simulink model "sampleModel7293_pp_1_1"  (R2018a)
settings: Solver=VariableStepAuto  StartTime=0.0  StopTime=10.0  RelTol=1e-3
undefined symbols (not defined in the file): DiscIntNeverNeededParam
libraries: simulink x367
(part 11 of 12)

== system sampleModel7293_pp_1_1/cfblk210/cfblk18 ==
  cfblk1 : Inport
  cfblk12 : Inport  Port=2
  cfblk13 : Inport  Port=3
  Action Port : ActionPort  ActionType=else
  cfblk10 : simulink/Discrete/Transfer Fcn First Order  PoleZ=0.95  ICPrevOutput=0.0  DoSatur=off
      settings: SourceProductName=Simulink
  cfblk11 : UnitDelay  SampleTime=-1
  cfblk3 : simulink/Discrete/Transfer Fcn Real Zero  ZeroZ=0.75  ICPrevInput=0.0  DoSatur=off
      settings: SourceProductName=Simulink  SourceProductBaseCode=SL
  cfblk4 : Subsystem  TreatAsAtomicUnit=on
  cfblk5 : DiscreteIntegrator  SampleTime=-1  OutDataTypeStr=double  ICPrevOutput=DiscIntNeverNeededParam  ICPrevScaledInput=DiscIntNeverNeededParam
  cfblk6 : DiscreteZeroPole  Poles=[0 0.5]  Gain=1  SampleTime=-1
  cfblk7 : DiscreteFir
  cfblk8 : UnitDelay  SampleTime=-1
  cfblk9 : Subsystem  TreatAsAtomicUnit=on
  cyemi_{1386..1394} (9 alike) : DataTypeConversion  OutDataTypeStr=double
  emi_1581 : Subsystem  TreatAsAtomicUnit=on
  emi_1583 : If  IfExpression=0 <= u1
  emi_1584 : DataTypeConversion  OutDataTypeStr=double
  emi_1688 : Subsystem  TreatAsAtomicUnit=on
  emi_1690 : If  IfExpression=0 <= u1
  emi_1691 : DataTypeConversion  OutDataTypeStr=double
  cfblk2 : Outport
  wires:
  cfblk3/1 -> cfblk2/1
  cyemi_1386/1 -> cfblk10/1
  cfblk5/1 -> cyemi_1386/1, emi_1584/1
  cyemi_1387/1 -> cfblk11/1
  cfblk8/1 -> cyemi_1387/1, emi_1691/1
  cyemi_1388/1 -> cfblk3/1
  cfblk13/1 -> cyemi_1388/1
  cyemi_1390/1 -> cfblk5/1
  cfblk11/1 -> cyemi_1390/1
  cyemi_1391/1 -> cfblk6/1
  cfblk12/1 -> cyemi_1391/1
  cyemi_1392/1 -> cfblk7/1
  cfblk1/1 -> cyemi_1392/1
  cyemi_1393/1 -> cfblk8/1
  cfblk6/1 -> cyemi_1394/1
  cyemi_1389/1 -> cfblk4/1(emi_1579)
  cfblk4/1(emi_1580) -> cyemi_1393/1
  emi_1583/1 -> cfblk4/Action
  emi_1583/2 -> emi_1581/Action
  emi_1584/1 -> emi_1583/1
  cyemi_1394/1 -> cfblk9/1(emi_1686)
  cfblk9/1(emi_1687) -> cyemi_1389/1
  emi_1690/1 -> cfblk9/Action
  emi_1690/2 -> emi_1688/Action
  emi_1691/1 -> emi_1690/1

== system sampleModel7293_pp_1_1/cfblk211/cfblk5 ==
  emi_1857 : Inport
  Action Port : ActionPort  ActionType=then
  cfblk5 : simulink/Discrete/Transfer Fcn First Order  PoleZ=0.95  ICPrevOutput=0.0  DoSatur=off
      settings: SourceProductName=Simulink
  emi_1858 : Outport
  wires:
  emi_1857/1 -> cfblk5/1
  cfblk5/1 -> emi_1858/1

== system sampleModel7293_pp_1_1/cfblk211/emi_1859 ==
  Action Port : ActionPort  ActionType=else
  emi_1860 : Assertion

== system sampleModel7293_pp_1_1/cfblk213/cfblk10 ==
  emi_1330 : Inport
  Action Port : ActionPort  ActionType=then
  cfblk10 : DiscreteFir
  emi_1331 : Outport
  wires:
  emi_1330/1 -> cfblk10/1
  cfblk10/1 -> emi_1331/1

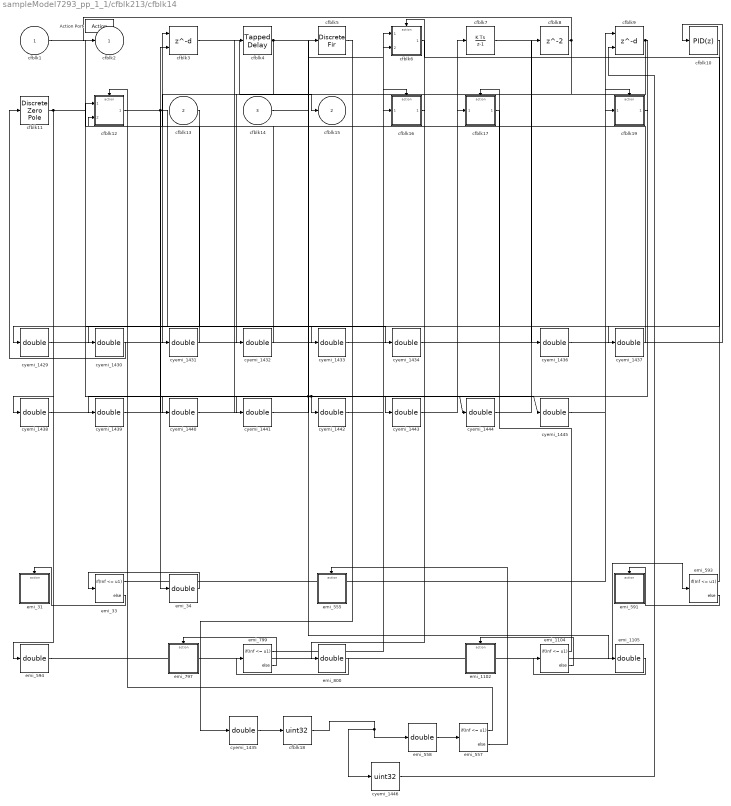
== system sampleModel7293_pp_1_1/cfblk213/cfblk14 ==
  cfblk1 : Inport
  cfblk13 : Inport  Port=2
  cfblk14 : Inport  Port=3
  Action Port : ActionPort  ActionType=then
  cfblk10 : simulink/Continuous/PID Controller  Controller=PID  TimeDomain=Discrete-time  SampleTime=-1  IntegratorMethod=Forward Euler  FilterMethod=Forward Euler  Form=Parallel  UseFilter=on  ControllerParametersSource=internal  P=1  I=1  D=0  N=100  InitialConditionSource=internal  InitialConditionForIntegrator=0  InitialConditionForFilter=0  ExternalReset=none  LimitOutput=off  UpperSaturationLimit=inf  LowerSaturationLimit=-inf  LinearizeAsGain=off  AntiWindupMode=none  Kb=1  TrackingMode=off  Kt=1  PParamMin=[]  PParamMax=[]  IParamMin=[]  IParamMax=[]  DParamMin=[]  DParamMax=[]  NParamMin=[]  NParamMax=[]  KbParamMin=[]  KbParamMax=[]  KtParamMin=[]  KtParamMax=[]  POutMin=[]  POutMax=[]  IOutMin=[]  IOutMax=[]  DOutMin=[]  DOutMax=[]  NOutMin=[]  NOutMax=[]  KbOutMin=[]  KbOutMax=[]  KtOutMin=[]  KtOutMax=[]  IntegratorOutMin=[]  IntegratorOutMax=[]  FilterOutMin=[]  FilterOutMax=[]  SumOutMin=[]  SumOutMax=[]  SumI1OutMin=[]  SumI1OutMax=[]  SumI2OutMin=[]  SumI2OutMax=[]  SumI3OutMin=[]  SumI3OutMax=[]  SumDOutMin=[]  SumDOutMax=[]  SaturationOutMin=[]  SaturationOutMax=[]  IntegratorContinuousStateAttributes=''  IntegratorStateMustResolveToSignalObject=off  IntegratorRTWStateStorageClass=Auto  FilterContinuousStateAttributes=''  FilterStateMustResolveToSignalObject=off  FilterRTWStateStorageClass=Auto  DifferentiatorICPrevScaledInput=0  DifferentiatorOutMin=[]  DifferentiatorOutMax=[]  FilterDiffOutCoefMin=[]  FilterDiffOutCoefMax=[]  SumDenOutMin=[]  SumDenOutMax=[]  SumNumOutMin=[]  SumNumOutMax=[]  ReciprocalOutMin=[]  ReciprocalOutMax=[]  DivideOutMin=[]  DivideOutMax=[]  TunerSelectOption=Transfer Function Based (PID Tuner App)
  cfblk11 : DiscreteZeroPole  Poles=[0 0.5]  Gain=1  SampleTime=-1
  cfblk12 : Subsystem  TreatAsAtomicUnit=on
  cfblk16 : Subsystem  TreatAsAtomicUnit=on
  cfblk17 : Subsystem  TreatAsAtomicUnit=on
  cfblk18 : DataTypeConversion  OutDataTypeStr=uint32
  cfblk19 : Subsystem  TreatAsAtomicUnit=on
  cfblk3 : Delay  DelayLengthSource=Input port
      settings: InputPortMap=u0,p1
  cfblk4 : simulink/Discrete/Tapped Delay  vinit=0.0  samptime=-1  NumDelays=1  DelayOrder=Oldest  includeCurrent=off
  cfblk5 : DiscreteFir
  cfblk6 : Subsystem  TreatAsAtomicUnit=on
  cfblk7 : DiscreteIntegrator  SampleTime=-1  OutDataTypeStr=double  ICPrevOutput=DiscIntNeverNeededParam  ICPrevScaledInput=DiscIntNeverNeededParam
  cfblk8 : Delay
  cfblk9 : Delay  DelayLengthSource=Input port
      settings: InputPortMap=u0,p1
  cyemi_{1429..1445} (17 alike) : DataTypeConversion  OutDataTypeStr=double
  cyemi_1446 : DataTypeConversion  OutDataTypeStr=uint32
  emi_1102 : Subsystem  TreatAsAtomicUnit=on
  emi_{33,557,593,799,1104} (5 alike) : If  IfExpression=Inf <= u1
  emi_{34,558,594,800,1105} (5 alike) : DataTypeConversion  OutDataTypeStr=double
  emi_31 : Subsystem  TreatAsAtomicUnit=on
  emi_555 : Subsystem  TreatAsAtomicUnit=on
  emi_591 : Subsystem  TreatAsAtomicUnit=on
  emi_797 : Subsystem  TreatAsAtomicUnit=on
  cfblk2 : Outport
  cfblk15 : Outport  Port=2
  wires:
  cfblk3/1 -> cfblk15/1
  cfblk8/1 -> cfblk2/1, emi_800/1
  cfblk1/1 -> cyemi_1442/1, cyemi_1444/1
  cfblk4/1 -> cyemi_1445/1, emi_1105/1, cyemi_1431/1
  cfblk9/1 -> cyemi_1432/1, cyemi_1437/1
  cyemi_1429/1 -> cfblk10/1
  cyemi_1430/1 -> cfblk11/1
  cfblk10/1 -> cyemi_1430/1
  cfblk11/1 -> cyemi_1434/1, emi_594/1
  cyemi_1435/1 -> cfblk18/1
  cfblk5/1 -> cyemi_1435/1
  cfblk7/1 -> cyemi_1436/1
  cyemi_1437/1 -> cfblk3/1
  cyemi_1438/1 -> cfblk3/2
  cfblk13/1 -> cyemi_1438/1
  cyemi_1439/1 -> cfblk4/1
  cyemi_1440/1 -> cfblk5/1
  cyemi_1443/1 -> cfblk7/1
  cfblk14/1 -> cyemi_1443/1
  cyemi_1444/1 -> cfblk8/1
  cyemi_1445/1 -> cfblk9/1
  cyemi_1446/1 -> cfblk9/2
  cfblk18/1 -> emi_558/1, cyemi_1446/1
  cyemi_1436/1 -> cfblk19/1(emi_29)
  cfblk19/1(emi_30) -> cyemi_1440/1
  emi_33/1 -> cfblk19/Action
  emi_33/2 -> emi_31/Action
  emi_34/1 -> emi_33/1
  cyemi_1431/1 -> cfblk12/1(emi_552)
  cyemi_1432/1 -> cfblk12/2(emi_553)
  cfblk12/1(emi_554) -> emi_34/1, cyemi_1433/1
  emi_557/1 -> cfblk12/Action
  emi_557/2 -> emi_555/Action
  emi_558/1 -> emi_557/1
  cyemi_1441/1 -> cfblk6/1(emi_588)
  cyemi_1442/1 -> cfblk6/2(emi_589)
  cfblk6/1(emi_590) -> cyemi_1439/1
  emi_593/1 -> cfblk6/Action
  emi_593/2 -> emi_591/Action
  emi_594/1 -> emi_593/1
  cyemi_1433/1 -> cfblk16/1(emi_795)
  cfblk16/1(emi_796) -> cyemi_1441/1
  emi_799/1 -> cfblk16/Action
  emi_799/2 -> emi_797/Action
  emi_800/1 -> emi_799/1
  cyemi_1434/1 -> cfblk17/1(emi_1100)
  cfblk17/1(emi_1101) -> cyemi_1429/1
  emi_1104/1 -> cfblk17/Action
  emi_1104/2 -> emi_1102/Action
  emi_1105/1 -> emi_1104/1

== system sampleModel7293_pp_1_1/cfblk213/cfblk15 ==
  cfblk1 : Inport
  cfblk9 : Inport  Port=2
  Action Port : ActionPort  ActionType=else
  cfblk11 : Delay
  cfblk12 : Delay
  cfblk3 : DiscreteIntegrator  SampleTime=-1  OutDataTypeStr=double  ICPrevOutput=DiscIntNeverNeededParam  ICPrevScaledInput=DiscIntNeverNeededParam
  cfblk4 : UnitDelay  SampleTime=-1
  cfblk5 : Delay
  cfblk6 : UnitDelay  SampleTime=-1
  cfblk7 : simulink/Discrete/Tapped Delay  vinit=0.0  samptime=-1  NumDelays=1  DelayOrder=Oldest  includeCurrent=off
  cfblk8 : DiscreteZeroPole  Poles=[0 0.5]  Gain=1  SampleTime=-1
  cyemi_{1449..1456} (8 alike) : DataTypeConversion  OutDataTypeStr=double
  cfblk2 : Outport
  cfblk10 : Outport  Port=2
  wires:
  cfblk1/1 -> cfblk10/1
  cfblk8/1 -> cfblk2/1
  cyemi_1449/1 -> cfblk11/1
  cfblk6/1 -> cyemi_1449/1
  cyemi_1450/1 -> cfblk12/1
  cfblk5/1 -> cyemi_1450/1
  cyemi_1451/1 -> cfblk3/1
  cfblk11/1 -> cyemi_1451/1
  cyemi_1452/1 -> cfblk4/1
  cfblk12/1 -> cyemi_1452/1
  cyemi_1453/1 -> cfblk5/1
  cfblk4/1 -> cyemi_1453/1
  cyemi_1454/1 -> cfblk6/1
  cfblk3/1 -> cyemi_1454/1
  cyemi_1455/1 -> cfblk7/1
  cfblk9/1 -> cyemi_1455/1
  cyemi_1456/1 -> cfblk8/1
  cfblk7/1 -> cyemi_1456/1

== system sampleModel7293_pp_1_1/cfblk213/cfblk16 ==
  emi_1358 : Inport
  Action Port : ActionPort  ActionType=then
  cfblk16 : Delay
  emi_1359 : Outport
  wires:
  emi_1358/1 -> cfblk16/1
  cfblk16/1 -> emi_1359/1

== system sampleModel7293_pp_1_1/cfblk213/emi_1332 ==
  Action Port : ActionPort  ActionType=else
  emi_1333 : Assertion

== system sampleModel7293_pp_1_1/cfblk213/emi_1360 ==
  Action Port : ActionPort  ActionType=else
  emi_1361 : Assertion

== system sampleModel7293_pp_1_1/cfblk165/cfblk15/cfblk11 ==
  emi_1022 : Inport
  Action Port : ActionPort  ActionType=then
  cfblk11 : DiscreteFir
  emi_1023 : Outport
  wires:
  emi_1022/1 -> cfblk11/1
  cfblk11/1 -> emi_1023/1

== system sampleModel7293_pp_1_1/cfblk165/cfblk15/cfblk12 ==
  emi_1408 : Inport
  Action Port : ActionPort  ActionType=then
  cfblk12 : Delay
  emi_1409 : Outport
  wires:
  emi_1408/1 -> cfblk12/1
  cfblk12/1 -> emi_1409/1

== system sampleModel7293_pp_1_1/cfblk165/cfblk15/cfblk13 ==
  emi_1764 : Inport
  Action Port : ActionPort  ActionType=then
  cfblk13 : DiscreteStateSpace  SampleTime=-1
  emi_1765 : Outport
  wires:
  emi_1764/1 -> cfblk13/1
  cfblk13/1 -> emi_1765/1

== system sampleModel7293_pp_1_1/cfblk165/cfblk15/emi_1024 ==
  Action Port : ActionPort  ActionType=else
  emi_1025 : Assertion

== system sampleModel7293_pp_1_1/cfblk165/cfblk15/emi_1410 ==
  Action Port : ActionPort  ActionType=else
  emi_1411 : Assertion

== system sampleModel7293_pp_1_1/cfblk165/cfblk15/emi_1766 ==
  Action Port : ActionPort  ActionType=else
  emi_1767 : Assertion

== system sampleModel7293_pp_1_1/cfblk165/cfblk16/cfblk11 ==
  emi_150 : Inport
  Action Port : ActionPort  ActionType=then
  cfblk11 : simulink/Discrete/Transfer Fcn Real Zero  ZeroZ=0.75  ICPrevInput=0.0  DoSatur=off
      settings: SourceProductName=Simulink  SourceProductBaseCode=SL
  emi_151 : Outport
  wires:
  emi_150/1 -> cfblk11/1
  cfblk11/1 -> emi_151/1

== system sampleModel7293_pp_1_1/cfblk165/cfblk16/cfblk12 ==
  emi_1157 : Inport
  emi_1158 : Inport  Port=2
  Action Port : ActionPort  ActionType=then
  cfblk12 : Delay  ShowEnablePort=on
      settings: InputPortMap=u0,e6
  emi_1159 : Outport
  wires:
  emi_1157/1 -> cfblk12/1
  emi_1158/1 -> cfblk12/2
  cfblk12/1 -> emi_1159/1

== system sampleModel7293_pp_1_1/cfblk165/cfblk16/cfblk8 ==
  emi_2075 : Inport
  Action Port : ActionPort  ActionType=then
  cfblk8 : UnitDelay  SampleTime=-1
  emi_2076 : Outport
  wires:
  emi_2075/1 -> cfblk8/1
  cfblk8/1 -> emi_2076/1

== system sampleModel7293_pp_1_1/cfblk165/cfblk16/emi_1160 ==
  Action Port : ActionPort  ActionType=else
  emi_1161 : Assertion

== system sampleModel7293_pp_1_1/cfblk165/cfblk16/emi_152 ==
  Action Port : ActionPort  ActionType=else
  emi_153 : Assertion

== system sampleModel7293_pp_1_1/cfblk165/cfblk16/emi_2077 ==
  Action Port : ActionPort  ActionType=else
  emi_2078 : Assertion

== system sampleModel7293_pp_1_1/cfblk167/cfblk17/cfblk5 ==
  emi_415 : Inport
  Action Port : ActionPort  ActionType=then
  cfblk5 : simulink/Discrete/Transfer Fcn Real Zero  ZeroZ=0.75  ICPrevInput=0.0  DoSatur=off
      settings: SourceProductName=Simulink  SourceProductBaseCode=SL
  emi_416 : Outport
  wires:
  emi_415/1 -> cfblk5/1
  cfblk5/1 -> emi_416/1

== system sampleModel7293_pp_1_1/cfblk167/cfblk17/cfblk7 ==
  emi_531 : Inport
  Action Port : ActionPort  ActionType=then
  cfblk7 : simulink/Continuous/PID Controller  Controller=PID  TimeDomain=Discrete-time  SampleTime=-1  IntegratorMethod=Forward Euler  FilterMethod=Forward Euler  Form=Parallel  UseFilter=on  ControllerParametersSource=internal  P=1  I=1  D=0  N=100  InitialConditionSource=internal  InitialConditionForIntegrator=0  InitialConditionForFilter=0  ExternalReset=none  LimitOutput=off  UpperSaturationLimit=inf  LowerSaturationLimit=-inf  LinearizeAsGain=off  AntiWindupMode=none  Kb=1  TrackingMode=off  Kt=1  PParamMin=[]  PParamMax=[]  IParamMin=[]  IParamMax=[]  DParamMin=[]  DParamMax=[]  NParamMin=[]  NParamMax=[]  KbParamMin=[]  KbParamMax=[]  KtParamMin=[]  KtParamMax=[]  POutMin=[]  POutMax=[]  IOutMin=[]  IOutMax=[]  DOutMin=[]  DOutMax=[]  NOutMin=[]  NOutMax=[]  KbOutMin=[]  KbOutMax=[]  KtOutMin=[]  KtOutMax=[]  IntegratorOutMin=[]  IntegratorOutMax=[]  FilterOutMin=[]  FilterOutMax=[]  SumOutMin=[]  SumOutMax=[]  SumI1OutMin=[]  SumI1OutMax=[]  SumI2OutMin=[]  SumI2OutMax=[]  SumI3OutMin=[]  SumI3OutMax=[]  SumDOutMin=[]  SumDOutMax=[]  SaturationOutMin=[]  SaturationOutMax=[]  IntegratorContinuousStateAttributes=''  IntegratorStateMustResolveToSignalObject=off  IntegratorRTWStateStorageClass=Auto  FilterContinuousStateAttributes=''  FilterStateMustResolveToSignalObject=off  FilterRTWStateStorageClass=Auto  DifferentiatorICPrevScaledInput=0  DifferentiatorOutMin=[]  DifferentiatorOutMax=[]  FilterDiffOutCoefMin=[]  FilterDiffOutCoefMax=[]  SumDenOutMin=[]  SumDenOutMax=[]  SumNumOutMin=[]  SumNumOutMax=[]  ReciprocalOutMin=[]  ReciprocalOutMax=[]  DivideOutMin=[]  DivideOutMax=[]  TunerSelectOption=Transfer Function Based (PID Tuner App)
  emi_532 : Outport
  wires:
  emi_531/1 -> cfblk7/1
  cfblk7/1 -> emi_532/1

== system sampleModel7293_pp_1_1/cfblk167/cfblk17/emi_417 ==
  Action Port : ActionPort  ActionType=else
  emi_418 : Assertion

== system sampleModel7293_pp_1_1/cfblk167/cfblk17/emi_533 ==
  Action Port : ActionPort  ActionType=else
  emi_534 : Assertion

== system sampleModel7293_pp_1_1/cfblk167/cfblk18/cfblk4 ==
  emi_1557 : Inport
  Action Port : ActionPort  ActionType=then
  cfblk4 : DiscreteZeroPole  Poles=[0 0.5]  Gain=1  SampleTime=-1
  emi_1558 : Outport
  wires:
  emi_1557/1 -> cfblk4/1
  cfblk4/1 -> emi_1558/1

== system sampleModel7293_pp_1_1/cfblk167/cfblk18/cfblk6 ==
  emi_2119 : Inport
  Action Port : ActionPort  ActionType=then
  cfblk6 : simulink/Discrete/Transfer Fcn Real Zero  ZeroZ=0.75  ICPrevInput=0.0  DoSatur=off
      settings: SourceProductName=Simulink  SourceProductBaseCode=SL
  emi_2120 : Outport
  wires:
  emi_2119/1 -> cfblk6/1
  cfblk6/1 -> emi_2120/1

== system sampleModel7293_pp_1_1/cfblk167/cfblk18/cfblk8 ==
  emi_36 : Inport
  Action Port : ActionPort  ActionType=then
  cfblk8 : DiscreteTransferFcn
  emi_37 : Outport
  wires:
  emi_36/1 -> cfblk8/1
  cfblk8/1 -> emi_37/1

== system sampleModel7293_pp_1_1/cfblk167/cfblk18/emi_1559 ==
  Action Port : ActionPort  ActionType=else
  emi_1560 : Assertion

== system sampleModel7293_pp_1_1/cfblk167/cfblk18/emi_2121 ==
  Action Port : ActionPort  ActionType=else
  emi_2122 : Assertion

== system sampleModel7293_pp_1_1/cfblk167/cfblk18/emi_38 ==
  Action Port : ActionPort  ActionType=else
  emi_39 : Assertion

== system sampleModel7293_pp_1_1/cfblk167/cfblk20/cfblk5 ==
  emi_72 : Inport
  Action Port : ActionPort  ActionType=then
  cfblk5 : simulink/Continuous/PID Controller  Controller=PID  TimeDomain=Discrete-time  SampleTime=-1  IntegratorMethod=Forward Euler  FilterMethod=Forward Euler  Form=Parallel  UseFilter=on  ControllerParametersSource=internal  P=1  I=1  D=0  N=100  InitialConditionSource=internal  InitialConditionForIntegrator=0  InitialConditionForFilter=0  ExternalReset=none  LimitOutput=off  UpperSaturationLimit=inf  LowerSaturationLimit=-inf  LinearizeAsGain=off  AntiWindupMode=none  Kb=1  TrackingMode=off  Kt=1  PParamMin=[]  PParamMax=[]  IParamMin=[]  IParamMax=[]  DParamMin=[]  DParamMax=[]  NParamMin=[]  NParamMax=[]  KbParamMin=[]  KbParamMax=[]  KtParamMin=[]  KtParamMax=[]  POutMin=[]  POutMax=[]  IOutMin=[]  IOutMax=[]  DOutMin=[]  DOutMax=[]  NOutMin=[]  NOutMax=[]  KbOutMin=[]  KbOutMax=[]  KtOutMin=[]  KtOutMax=[]  IntegratorOutMin=[]  IntegratorOutMax=[]  FilterOutMin=[]  FilterOutMax=[]  SumOutMin=[]  SumOutMax=[]  SumI1OutMin=[]  SumI1OutMax=[]  SumI2OutMin=[]  SumI2OutMax=[]  SumI3OutMin=[]  SumI3OutMax=[]  SumDOutMin=[]  SumDOutMax=[]  SaturationOutMin=[]  SaturationOutMax=[]  IntegratorContinuousStateAttributes=''  IntegratorStateMustResolveToSignalObject=off  IntegratorRTWStateStorageClass=Auto  FilterContinuousStateAttributes=''  FilterStateMustResolveToSignalObject=off  FilterRTWStateStorageClass=Auto  DifferentiatorICPrevScaledInput=0  DifferentiatorOutMin=[]  DifferentiatorOutMax=[]  FilterDiffOutCoefMin=[]  FilterDiffOutCoefMax=[]  SumDenOutMin=[]  SumDenOutMax=[]  SumNumOutMin=[]  SumNumOutMax=[]  ReciprocalOutMin=[]  ReciprocalOutMax=[]  DivideOutMin=[]  DivideOutMax=[]  TunerSelectOption=Transfer Function Based (PID Tuner App)
  emi_73 : Outport
  wires:
  emi_72/1 -> cfblk5/1
  cfblk5/1 -> emi_73/1

== system sampleModel7293_pp_1_1/cfblk167/cfblk20/cfblk8 ==
  emi_250 : Inport
  Action Port : ActionPort  ActionType=then
  cfblk8 : Delay
  emi_251 : Outport
  wires:
  emi_250/1 -> cfblk8/1
  cfblk8/1 -> emi_251/1

== system sampleModel7293_pp_1_1/cfblk167/cfblk20/emi_252 ==
  Action Port : ActionPort  ActionType=else
  emi_253 : Assertion

== system sampleModel7293_pp_1_1/cfblk167/cfblk20/emi_74 ==
  Action Port : ActionPort  ActionType=else
  emi_75 : Assertion

== system sampleModel7293_pp_1_1/cfblk170/cfblk14/cfblk5 ==
  emi_1664 : Inport
  emi_1665 : Inport  Port=2
  Action Port : ActionPort  ActionType=then
  cfblk5 : Delay  ShowEnablePort=on
      settings: InputPortMap=u0,e6
  emi_1666 : Outport
  wires:
  emi_1664/1 -> cfblk5/1
  emi_1665/1 -> cfblk5/2
  cfblk5/1 -> emi_1666/1

== system sampleModel7293_pp_1_1/cfblk170/cfblk14/cfblk8 ==
  emi_667 : Inport
  Action Port : ActionPort  ActionType=then
  cfblk8 : Delay
  emi_668 : Outport
  wires:
  emi_667/1 -> cfblk8/1
  cfblk8/1 -> emi_668/1

== system sampleModel7293_pp_1_1/cfblk170/cfblk14/emi_1667 ==
  Action Port : ActionPort  ActionType=else
  emi_1668 : Assertion

== system sampleModel7293_pp_1_1/cfblk170/cfblk14/emi_669 ==
  Action Port : ActionPort  ActionType=else
  emi_670 : Assertion

== system sampleModel7293_pp_1_1/cfblk170/cfblk15/cfblk4 ==
  emi_1864 : Inport
  Action Port : ActionPort  ActionType=then
  cfblk4 : DiscreteFir
  emi_1865 : Outport
  wires:
  emi_1864/1 -> cfblk4/1
  cfblk4/1 -> emi_1865/1

== system sampleModel7293_pp_1_1/cfblk170/cfblk15/cfblk5 ==
  emi_1843 : Inport
  Action Port : ActionPort  ActionType=then
  cfblk5 : Delay
  emi_1844 : Outport
  wires:
  emi_1843/1 -> cfblk5/1
  cfblk5/1 -> emi_1844/1

== system sampleModel7293_pp_1_1/cfblk170/cfblk15/cfblk7 ==
  emi_185 : Inport
  emi_186 : Inport  Port=2
  Action Port : ActionPort  ActionType=then
  cfblk7 : simulink/Continuous/PID Controller (2DOF)  Controller=PID  TimeDomain=Discrete-time  SampleTime=-1  IntegratorMethod=Forward Euler  FilterMethod=Forward Euler  Form=Parallel  UseFilter=on  ControllerParametersSource=internal  P=1  I=1  D=0  N=100  b=1  c=1  InitialConditionSource=internal  InitialConditionForIntegrator=0  InitialConditionForFilter=0  ExternalReset=none  LimitOutput=off  UpperSaturationLimit=inf  LowerSaturationLimit=-inf  LinearizeAsGain=off  AntiWindupMode=none  Kb=1  TrackingMode=off  Kt=1  PParamMin=[]  PParamMax=[]  IParamMin=[]  IParamMax=[]  DParamMin=[]  DParamMax=[]  NParamMin=[]  NParamMax=[]  bParamMin=[]  bParamMax=[]  cParamMin=[]  cParamMax=[]  KbParamMin=[]  KbParamMax=[]  KtParamMin=[]  KtParamMax=[]  POutMin=[]  POutMax=[]  IOutMin=[]  IOutMax=[]  DOutMin=[]  DOutMax=[]  NOutMin=[]  NOutMax=[]  bOutMin=[]  bOutMax=[]  cOutMin=[]  cOutMax=[]  KbOutMin=[]  KbOutMax=[]  KtOutMin=[]  KtOutMax=[]  IntegratorOutMin=[]  IntegratorOutMax=[]  FilterOutMin=[]  FilterOutMax=[]  SumOutMin=[]  SumOutMax=[]  Sum1OutMin=[]  Sum1OutMax=[]  Sum2OutMin=[]  Sum2OutMax=[]  Sum3OutMin=[]  Sum3OutMax=[]  SumI1OutMin=[]  SumI1OutMax=[]  SumI2OutMin=[]  SumI2OutMax=[]  SumI3OutMin=[]  SumI3OutMax=[]  SumDOutMin=[]  SumDOutMax=[]  SaturationOutMin=[]  SaturationOutMax=[]  IntegratorContinuousStateAttributes=''  IntegratorStateMustResolveToSignalObject=off  IntegratorRTWStateStorageClass=Auto  FilterContinuousStateAttributes=''  FilterStateMustResolveToSignalObject=off  FilterRTWStateStorageClass=Auto  DifferentiatorICPrevScaledInput=0  DifferentiatorOutMin=[]  DifferentiatorOutMax=[]  FilterDiffOutCoefMin=[]  FilterDiffOutCoefMax=[]  SumDenOutMin=[]  SumDenOutMax=[]  SumNumOutMin=[]  SumNumOutMax=[]  ReciprocalOutMin=[]  ReciprocalOutMax=[]  DivideOutMin=[]  DivideOutMax=[]  TunerSelectOption=Transfer Function Based (PID Tuner App)
  emi_187 : Outport
  wires:
  emi_185/1 -> cfblk7/1
  emi_186/1 -> cfblk7/2
  cfblk7/1 -> emi_187/1

== system sampleModel7293_pp_1_1/cfblk170/cfblk15/emi_1845 ==
  Action Port : ActionPort  ActionType=else
  emi_1846 : Assertion

== system sampleModel7293_pp_1_1/cfblk170/cfblk15/emi_1866 ==
  Action Port : ActionPort  ActionType=else
  emi_1867 : Assertion

== system sampleModel7293_pp_1_1/cfblk170/cfblk15/emi_188 ==
  Action Port : ActionPort  ActionType=else
  emi_189 : Assertion

== system sampleModel7293_pp_1_1/cfblk170/cfblk16/cfblk3 ==
  emi_1636 : Inport
  Action Port : ActionPort  ActionType=then
  cfblk3 : simulink/Discrete/Transfer Fcn Real Zero  ZeroZ=0.75  ICPrevInput=0.0  DoSatur=off
      settings: SourceProductName=Simulink  SourceProductBaseCode=SL
  emi_1637 : Outport
  wires:
  emi_1636/1 -> cfblk3/1
  cfblk3/1 -> emi_1637/1

== system sampleModel7293_pp_1_1/cfblk170/cfblk16/emi_1638 ==
  Action Port : ActionPort  ActionType=else
  emi_1639 : Assertion

== system sampleModel7293_pp_1_1/cfblk170/cfblk17/cfblk3 ==
  emi_1629 : Inport
  Action Port : ActionPort  ActionType=then
  cfblk3 : simulink/Discrete/Transfer Fcn Real Zero  ZeroZ=0.75  ICPrevInput=0.0  DoSatur=off
      settings: SourceProductName=Simulink  SourceProductBaseCode=SL
  emi_1630 : Outport
  wires:
  emi_1629/1 -> cfblk3/1
  cfblk3/1 -> emi_1630/1

== system sampleModel7293_pp_1_1/cfblk170/cfblk17/emi_1631 ==
  Action Port : ActionPort  ActionType=else
  emi_1632 : Assertion

== system sampleModel7293_pp_1_1/cfblk171/cfblk10/cfblk11 ==
  emi_1172 : Inport
  emi_1173 : Inport  Port=2
  Action Port : ActionPort  ActionType=then
  cfblk11 : Delay  ShowEnablePort=on
      settings: InputPortMap=u0,e6
  emi_1174 : Outport
  wires:
  emi_1172/1 -> cfblk11/1
  emi_1173/1 -> cfblk11/2
  cfblk11/1 -> emi_1174/1

== system sampleModel7293_pp_1_1/cfblk171/cfblk10/cfblk12 ==
  emi_889 : Inport
  Action Port : ActionPort  ActionType=then
  cfblk12 : simulink/Discrete/Tapped Delay  vinit=0.0  samptime=-1  NumDelays=1  DelayOrder=Oldest  includeCurrent=off
  emi_890 : Outport
  wires:
  emi_889/1 -> cfblk12/1
  cfblk12/1 -> emi_890/1

== system sampleModel7293_pp_1_1/cfblk171/cfblk10/cfblk13 ==
  emi_2047 : Inport
  Action Port : ActionPort  ActionType=then
  cfblk13 : Delay
  emi_2048 : Outport
  wires:
  emi_2047/1 -> cfblk13/1
  cfblk13/1 -> emi_2048/1

== system sampleModel7293_pp_1_1/cfblk171/cfblk10/cfblk5 ==
  emi_560 : Inport
  Action Port : ActionPort  ActionType=then
  cfblk5 : simulink/Discrete/Transfer Fcn Lead or Lag  PoleZ=0.95  ZeroZ=0.75  ICPrevOutput=0.0  ICPrevInput=0.0  DoSatur=off
      settings: SourceProductName=Simulink  SourceProductBaseCode=SL
  emi_561 : Outport
  wires:
  emi_560/1 -> cfblk5/1
  cfblk5/1 -> emi_561/1

== system sampleModel7293_pp_1_1/cfblk171/cfblk10/cfblk6 ==
  emi_1386 : Inport
  Action Port : ActionPort  ActionType=then
  cfblk6 : UnitDelay  SampleTime=-1
  emi_1387 : Outport
  wires:
  emi_1386/1 -> cfblk6/1
  cfblk6/1 -> emi_1387/1

== system sampleModel7293_pp_1_1/cfblk171/cfblk10/emi_1175 ==
  Action Port : ActionPort  ActionType=else
  emi_1176 : Assertion

== system sampleModel7293_pp_1_1/cfblk171/cfblk10/emi_1388 ==
  Action Port : ActionPort  ActionType=else
  emi_1389 : Assertion

== system sampleModel7293_pp_1_1/cfblk171/cfblk10/emi_2049 ==
  Action Port : ActionPort  ActionType=else
  emi_2050 : Assertion

== system sampleModel7293_pp_1_1/cfblk171/cfblk10/emi_562 ==
  Action Port : ActionPort  ActionType=else
  emi_563 : Assertion

== system sampleModel7293_pp_1_1/cfblk171/cfblk10/emi_891 ==
  Action Port : ActionPort  ActionType=else
  emi_892 : Assertion

== system sampleModel7293_pp_1_1/cfblk173/cfblk13/cfblk10 ==
  emi_1714 : Inport
  Action Port : ActionPort  ActionType=then
  cfblk10 : DiscreteStateSpace  SampleTime=-1
  emi_1715 : Outport
  wires:
  emi_1714/1 -> cfblk10/1
  cfblk10/1 -> emi_1715/1

== system sampleModel7293_pp_1_1/cfblk173/cfblk13/cfblk9 ==
  emi_1071 : Inport
  Action Port : ActionPort  ActionType=then
  cfblk9 : simulink/Discrete/Transfer Fcn Lead or Lag  PoleZ=0.95  ZeroZ=0.75  ICPrevOutput=0.0  ICPrevInput=0.0  DoSatur=off
      settings: SourceProductName=Simulink  SourceProductBaseCode=SL
  emi_1072 : Outport
  wires:
  emi_1071/1 -> cfblk9/1
  cfblk9/1 -> emi_1072/1

== system sampleModel7293_pp_1_1/cfblk173/cfblk13/emi_1073 ==
  Action Port : ActionPort  ActionType=else
  emi_1074 : Assertion

== system sampleModel7293_pp_1_1/cfblk173/cfblk13/emi_1716 ==
  Action Port : ActionPort  ActionType=else
  emi_1717 : Assertion

== system sampleModel7293_pp_1_1/cfblk173/cfblk14/cfblk3 ==
  emi_839 : Inport
  Action Port : ActionPort  ActionType=then
  cfblk3 : DiscreteTransferFcn
  emi_840 : Outport
  wires:
  emi_839/1 -> cfblk3/1
  cfblk3/1 -> emi_840/1

== system sampleModel7293_pp_1_1/cfblk173/cfblk14/cfblk4 ==
  emi_1983 : Inport
  emi_1984 : Inport  Port=2
  Action Port : ActionPort  ActionType=then
  cfblk4 : Delay  DelayLengthSource=Input port
      settings: InputPortMap=u0,p1
  emi_1985 : Outport
  wires:
  emi_1983/1 -> cfblk4/1
  emi_1984/1 -> cfblk4/2
  cfblk4/1 -> emi_1985/1

== system sampleModel7293_pp_1_1/cfblk173/cfblk14/emi_1986 ==
  Action Port : ActionPort  ActionType=else
  emi_1987 : Assertion

== system sampleModel7293_pp_1_1/cfblk173/cfblk14/emi_841 ==
  Action Port : ActionPort  ActionType=else
  emi_842 : Assertion

== system sampleModel7293_pp_1_1/cfblk175/cfblk16/cfblk3 ==
  emi_1085 : Inport
  Action Port : ActionPort  ActionType=then
  cfblk3 : simulink/Discrete/Transfer Fcn First Order  PoleZ=0.95  ICPrevOutput=0.0  DoSatur=off
      settings: SourceProductName=Simulink
  emi_1086 : Outport
  wires:
  emi_1085/1 -> cfblk3/1
  cfblk3/1 -> emi_1086/1

== system sampleModel7293_pp_1_1/cfblk175/cfblk16/cfblk6 ==
  emi_1252 : Inport
  Action Port : ActionPort  ActionType=then
  cfblk6 : simulink/Discrete/Transfer Fcn First Order  PoleZ=0.95  ICPrevOutput=0.0  DoSatur=off
      settings: SourceProductName=Simulink
  emi_1253 : Outport
  wires:
  emi_1252/1 -> cfblk6/1
  cfblk6/1 -> emi_1253/1

== system sampleModel7293_pp_1_1/cfblk175/cfblk16/emi_1087 ==
  Action Port : ActionPort  ActionType=else
  emi_1088 : Assertion

== system sampleModel7293_pp_1_1/cfblk175/cfblk16/emi_1254 ==
  Action Port : ActionPort  ActionType=else
  emi_1255 : Assertion

== system sampleModel7293_pp_1_1/cfblk175/cfblk17/cfblk3 ==
  emi_272 : Inport
  Action Port : ActionPort  ActionType=then
  cfblk3 : simulink/Discrete/Tapped Delay  vinit=0.0  samptime=-1  NumDelays=1  DelayOrder=Oldest  includeCurrent=off
  emi_273 : Outport
  wires:
  emi_272/1 -> cfblk3/1
  cfblk3/1 -> emi_273/1

== system sampleModel7293_pp_1_1/cfblk175/cfblk17/cfblk5 ==
  emi_1486 : Inport
  Action Port : ActionPort  ActionType=then
  cfblk5 : simulink/Discrete/Tapped Delay  vinit=0.0  samptime=-1  NumDelays=1  DelayOrder=Oldest  includeCurrent=off
  emi_1487 : Outport
  wires:
  emi_1486/1 -> cfblk5/1
  cfblk5/1 -> emi_1487/1

== system sampleModel7293_pp_1_1/cfblk175/cfblk17/cfblk8 ==
  emi_2061 : Inport
  Action Port : ActionPort  ActionType=then
  cfblk8 : UnitDelay  SampleTime=-1
  emi_2062 : Outport
  wires:
  emi_2061/1 -> cfblk8/1
  cfblk8/1 -> emi_2062/1

== system sampleModel7293_pp_1_1/cfblk175/cfblk17/emi_1488 ==
  Action Port : ActionPort  ActionType=else
  emi_1489 : Assertion

== system sampleModel7293_pp_1_1/cfblk175/cfblk17/emi_2063 ==
  Action Port : ActionPort  ActionType=else
  emi_2064 : Assertion

== system sampleModel7293_pp_1_1/cfblk175/cfblk17/emi_274 ==
  Action Port : ActionPort  ActionType=else
  emi_275 : Assertion

== system sampleModel7293_pp_1_1/cfblk180/cfblk17/cfblk3 ==
  emi_817 : Inport
  emi_818 : Inport  Port=2
  Action Port : ActionPort  ActionType=then
  cfblk3 : simulink/Continuous/PID Controller (2DOF)  Controller=PID  TimeDomain=Discrete-time  SampleTime=-1  IntegratorMethod=Forward Euler  FilterMethod=Forward Euler  Form=Parallel  UseFilter=on  ControllerParametersSource=internal  P=1  I=1  D=0  N=100  b=1  c=1  InitialConditionSource=internal  InitialConditionForIntegrator=0  InitialConditionForFilter=0  ExternalReset=none  LimitOutput=off  UpperSaturationLimit=inf  LowerSaturationLimit=-inf  LinearizeAsGain=off  AntiWindupMode=none  Kb=1  TrackingMode=off  Kt=1  PParamMin=[]  PParamMax=[]  IParamMin=[]  IParamMax=[]  DParamMin=[]  DParamMax=[]  NParamMin=[]  NParamMax=[]  bParamMin=[]  bParamMax=[]  cParamMin=[]  cParamMax=[]  KbParamMin=[]  KbParamMax=[]  KtParamMin=[]  KtParamMax=[]  POutMin=[]  POutMax=[]  IOutMin=[]  IOutMax=[]  DOutMin=[]  DOutMax=[]  NOutMin=[]  NOutMax=[]  bOutMin=[]  bOutMax=[]  cOutMin=[]  cOutMax=[]  KbOutMin=[]  KbOutMax=[]  KtOutMin=[]  KtOutMax=[]  IntegratorOutMin=[]  IntegratorOutMax=[]  FilterOutMin=[]  FilterOutMax=[]  SumOutMin=[]  SumOutMax=[]  Sum1OutMin=[]  Sum1OutMax=[]  Sum2OutMin=[]  Sum2OutMax=[]  Sum3OutMin=[]  Sum3OutMax=[]  SumI1OutMin=[]  SumI1OutMax=[]  SumI2OutMin=[]  SumI2OutMax=[]  SumI3OutMin=[]  SumI3OutMax=[]  SumDOutMin=[]  SumDOutMax=[]  SaturationOutMin=[]  SaturationOutMax=[]  IntegratorContinuousStateAttributes=''  IntegratorStateMustResolveToSignalObject=off  IntegratorRTWStateStorageClass=Auto  FilterContinuousStateAttributes=''  FilterStateMustResolveToSignalObject=off  FilterRTWStateStorageClass=Auto  DifferentiatorICPrevScaledInput=0  DifferentiatorOutMin=[]  DifferentiatorOutMax=[]  FilterDiffOutCoefMin=[]  FilterDiffOutCoefMax=[]  SumDenOutMin=[]  SumDenOutMax=[]  SumNumOutMin=[]  SumNumOutMax=[]  ReciprocalOutMin=[]  ReciprocalOutMax=[]  DivideOutMin=[]  DivideOutMax=[]  TunerSelectOption=Transfer Function Based (PID Tuner App)
  emi_819 : Outport
  wires:
  emi_817/1 -> cfblk3/1
  emi_818/1 -> cfblk3/2
  cfblk3/1 -> emi_819/1

== system sampleModel7293_pp_1_1/cfblk180/cfblk17/cfblk5 ==
  emi_1927 : Inport
  Action Port : ActionPort  ActionType=then
  cfblk5 : simulink/Discrete/Tapped Delay  vinit=0.0  samptime=-1  NumDelays=1  DelayOrder=Oldest  includeCurrent=off
  emi_1928 : Outport
  wires:
  emi_1927/1 -> cfblk5/1
  cfblk5/1 -> emi_1928/1

== system sampleModel7293_pp_1_1/cfblk180/cfblk17/cfblk7 ==
  emi_1500 : Inport
  emi_1501 : Inport  Port=2
  Action Port : ActionPort  ActionType=then
  cfblk7 : simulink/Continuous/PID Controller (2DOF)  Controller=PID  TimeDomain=Discrete-time  SampleTime=-1  IntegratorMethod=Forward Euler  FilterMethod=Forward Euler  Form=Parallel  UseFilter=on  ControllerParametersSource=internal  P=1  I=1  D=0  N=100  b=1  c=1  InitialConditionSource=internal  InitialConditionForIntegrator=0  InitialConditionForFilter=0  ExternalReset=none  LimitOutput=off  UpperSaturationLimit=inf  LowerSaturationLimit=-inf  LinearizeAsGain=off  AntiWindupMode=none  Kb=1  TrackingMode=off  Kt=1  PParamMin=[]  PParamMax=[]  IParamMin=[]  IParamMax=[]  DParamMin=[]  DParamMax=[]  NParamMin=[]  NParamMax=[]  bParamMin=[]  bParamMax=[]  cParamMin=[]  cParamMax=[]  KbParamMin=[]  KbParamMax=[]  KtParamMin=[]  KtParamMax=[]  POutMin=[]  POutMax=[]  IOutMin=[]  IOutMax=[]  DOutMin=[]  DOutMax=[]  NOutMin=[]  NOutMax=[]  bOutMin=[]  bOutMax=[]  cOutMin=[]  cOutMax=[]  KbOutMin=[]  KbOutMax=[]  KtOutMin=[]  KtOutMax=[]  IntegratorOutMin=[]  IntegratorOutMax=[]  FilterOutMin=[]  FilterOutMax=[]  SumOutMin=[]  SumOutMax=[]  Sum1OutMin=[]  Sum1OutMax=[]  Sum2OutMin=[]  Sum2OutMax=[]  Sum3OutMin=[]  Sum3OutMax=[]  SumI1OutMin=[]  SumI1OutMax=[]  SumI2OutMin=[]  SumI2OutMax=[]  SumI3OutMin=[]  SumI3OutMax=[]  SumDOutMin=[]  SumDOutMax=[]  SaturationOutMin=[]  SaturationOutMax=[]  IntegratorContinuousStateAttributes=''  IntegratorStateMustResolveToSignalObject=off  IntegratorRTWStateStorageClass=Auto  FilterContinuousStateAttributes=''  FilterStateMustResolveToSignalObject=off  FilterRTWStateStorageClass=Auto  DifferentiatorICPrevScaledInput=0  DifferentiatorOutMin=[]  DifferentiatorOutMax=[]  FilterDiffOutCoefMin=[]  FilterDiffOutCoefMax=[]  SumDenOutMin=[]  SumDenOutMax=[]  SumNumOutMin=[]  SumNumOutMax=[]  ReciprocalOutMin=[]  ReciprocalOutMax=[]  DivideOutMin=[]  DivideOutMax=[]  TunerSelectOption=Transfer Function Based (PID Tuner App)
  emi_1502 : Outport
  wires:
  emi_1500/1 -> cfblk7/1
  emi_1501/1 -> cfblk7/2
  cfblk7/1 -> emi_1502/1

== system sampleModel7293_pp_1_1/cfblk180/cfblk17/cfblk8 ==
  emi_352 : Inport
  Action Port : ActionPort  ActionType=then
  cfblk8 : DiscreteFir
  emi_353 : Outport
  wires:
  emi_352/1 -> cfblk8/1
  cfblk8/1 -> emi_353/1

== system sampleModel7293_pp_1_1/cfblk180/cfblk17/cfblk9 ==
  emi_108 : Inport
  Action Port : ActionPort  ActionType=then
  cfblk9 : simulink/Discrete/Transfer Fcn Lead or Lag  PoleZ=0.95  ZeroZ=0.75  ICPrevOutput=0.0  ICPrevInput=0.0  DoSatur=off
      settings: SourceProductName=Simulink  SourceProductBaseCode=SL
  emi_109 : Outport
  wires:
  emi_108/1 -> cfblk9/1
  cfblk9/1 -> emi_109/1

== system sampleModel7293_pp_1_1/cfblk180/cfblk17/emi_110 ==
  Action Port : ActionPort  ActionType=else
  emi_111 : Assertion

== system sampleModel7293_pp_1_1/cfblk180/cfblk17/emi_1503 ==
  Action Port : ActionPort  ActionType=else
  emi_1504 : Assertion

== system sampleModel7293_pp_1_1/cfblk180/cfblk17/emi_1929 ==
  Action Port : ActionPort  ActionType=else
  emi_1930 : Assertion

== system sampleModel7293_pp_1_1/cfblk180/cfblk17/emi_354 ==
  Action Port : ActionPort  ActionType=else
  emi_355 : Assertion

== system sampleModel7293_pp_1_1/cfblk180/cfblk17/emi_820 ==
  Action Port : ActionPort  ActionType=else
  emi_821 : Assertion

== system sampleModel7293_pp_1_1/cfblk180/cfblk18/cfblk10 ==
  emi_2105 : Inport
  Action Port : ActionPort  ActionType=then
  cfblk10 : simulink/Discrete/Tapped Delay  vinit=0.0  samptime=-1  NumDelays=1  DelayOrder=Oldest  includeCurrent=off
  emi_2106 : Outport
  wires:
  emi_2105/1 -> cfblk10/1
  cfblk10/1 -> emi_2106/1

== system sampleModel7293_pp_1_1/cfblk180/cfblk18/cfblk5 ==
  emi_2082 : Inport
  emi_2083 : Inport  Port=2
  Action Port : ActionPort  ActionType=then
  cfblk5 : Delay  ShowEnablePort=on
      settings: InputPortMap=u0,e6
  emi_2084 : Outport
  wires:
  emi_2082/1 -> cfblk5/1
  emi_2083/1 -> cfblk5/2
  cfblk5/1 -> emi_2084/1

== system sampleModel7293_pp_1_1/cfblk180/cfblk18/cfblk7 ==
  emi_236 : Inport
  Action Port : ActionPort  ActionType=then
  cfblk7 : simulink/Discrete/Transfer Fcn Real Zero  ZeroZ=0.75  ICPrevInput=0.0  DoSatur=off
      settings: SourceProductName=Simulink  SourceProductBaseCode=SL
  emi_237 : Outport
  wires:
  emi_236/1 -> cfblk7/1
  cfblk7/1 -> emi_237/1

== system sampleModel7293_pp_1_1/cfblk180/cfblk18/emi_2085 ==
  Action Port : ActionPort  ActionType=else
  emi_2086 : Assertion

== system sampleModel7293_pp_1_1/cfblk180/cfblk18/emi_2107 ==
  Action Port : ActionPort  ActionType=else
  emi_2108 : Assertion

== system sampleModel7293_pp_1_1/cfblk180/cfblk18/emi_238 ==
  Action Port : ActionPort  ActionType=else
  emi_239 : Assertion

== system sampleModel7293_pp_1_1/cfblk182/cfblk12/cfblk3 ==
  emi_980 : Inport
  Action Port : ActionPort  ActionType=then
  cfblk3 : simulink/Discrete/Transfer Fcn Lead or Lag  PoleZ=0.95  ZeroZ=0.75  ICPrevOutput=0.0  ICPrevInput=0.0  DoSatur=off
      settings: SourceProductName=Simulink  SourceProductBaseCode=SL
  emi_981 : Outport
  wires:
  emi_980/1 -> cfblk3/1
  cfblk3/1 -> emi_981/1

== system sampleModel7293_pp_1_1/cfblk182/cfblk12/cfblk7 ==
  emi_101 : Inport
  Action Port : ActionPort  ActionType=then
  cfblk7 : simulink/Discrete/Transfer Fcn Lead or Lag  PoleZ=0.95  ZeroZ=0.75  ICPrevOutput=0.0  ICPrevInput=0.0  DoSatur=off
      settings: SourceProductName=Simulink  SourceProductBaseCode=SL
  emi_102 : Outport
  wires:
  emi_101/1 -> cfblk7/1
  cfblk7/1 -> emi_102/1

== system sampleModel7293_pp_1_1/cfblk182/cfblk12/emi_103 ==
  Action Port : ActionPort  ActionType=else
  emi_104 : Assertion

== system sampleModel7293_pp_1_1/cfblk182/cfblk12/emi_982 ==
  Action Port : ActionPort  ActionType=else
  emi_983 : Assertion

== system sampleModel7293_pp_1_1/cfblk182/cfblk13/cfblk11 ==
  emi_1464 : Inport
  Action Port : ActionPort  ActionType=then
  cfblk11 : Delay
  emi_1465 : Outport
  wires:
  emi_1464/1 -> cfblk11/1
  cfblk11/1 -> emi_1465/1

== system sampleModel7293_pp_1_1/cfblk182/cfblk13/cfblk3 ==
  emi_1672 : Inport
  Action Port : ActionPort  ActionType=then
  cfblk3 : simulink/Discrete/Transfer Fcn First Order  PoleZ=0.95  ICPrevOutput=0.0  DoSatur=off
      settings: SourceProductName=Simulink
  emi_1673 : Outport
  wires:
  emi_1672/1 -> cfblk3/1
  cfblk3/1 -> emi_1673/1

== system sampleModel7293_pp_1_1/cfblk182/cfblk13/emi_1466 ==
  Action Port : ActionPort  ActionType=else
  emi_1467 : Assertion

== system sampleModel7293_pp_1_1/cfblk182/cfblk13/emi_1674 ==
  Action Port : ActionPort  ActionType=else
  emi_1675 : Assertion

== system sampleModel7293_pp_1_1/cfblk184/cfblk16/cfblk12 ==
  emi_408 : Inport
  Action Port : ActionPort  ActionType=then
  cfblk12 : Delay
  emi_409 : Outport
  wires:
  emi_408/1 -> cfblk12/1
  cfblk12/1 -> emi_409/1

== system sampleModel7293_pp_1_1/cfblk184/cfblk16/cfblk13 ==
  emi_1064 : Inport
  Action Port : ActionPort  ActionType=then
  cfblk13 : simulink/Discrete/Tapped Delay  vinit=0.0  samptime=-1  NumDelays=1  DelayOrder=Oldest  includeCurrent=off
  emi_1065 : Outport
  wires:
  emi_1064/1 -> cfblk13/1
  cfblk13/1 -> emi_1065/1

== system sampleModel7293_pp_1_1/cfblk184/cfblk16/cfblk4 ==
  emi_1001 : Inport
  Action Port : ActionPort  ActionType=then
  cfblk4 : simulink/Discrete/Tapped Delay  vinit=0.0  samptime=-1  NumDelays=1  DelayOrder=Oldest  includeCurrent=off
  emi_1002 : Outport
  wires:
  emi_1001/1 -> cfblk4/1
  cfblk4/1 -> emi_1002/1

== system sampleModel7293_pp_1_1/cfblk184/cfblk16/cfblk5 ==
  emi_1092 : Inport
  emi_1093 : Inport  Port=2
  Action Port : ActionPort  ActionType=then
  cfblk5 : simulink/Continuous/PID Controller (2DOF)  Controller=PID  TimeDomain=Discrete-time  SampleTime=-1  IntegratorMethod=Forward Euler  FilterMethod=Forward Euler  Form=Parallel  UseFilter=on  ControllerParametersSource=internal  P=1  I=1  D=0  N=100  b=1  c=1  InitialConditionSource=internal  InitialConditionForIntegrator=0  InitialConditionForFilter=0  ExternalReset=none  LimitOutput=off  UpperSaturationLimit=inf  LowerSaturationLimit=-inf  LinearizeAsGain=off  AntiWindupMode=none  Kb=1  TrackingMode=off  Kt=1  PParamMin=[]  PParamMax=[]  IParamMin=[]  IParamMax=[]  DParamMin=[]  DParamMax=[]  NParamMin=[]  NParamMax=[]  bParamMin=[]  bParamMax=[]  cParamMin=[]  cParamMax=[]  KbParamMin=[]  KbParamMax=[]  KtParamMin=[]  KtParamMax=[]  POutMin=[]  POutMax=[]  IOutMin=[]  IOutMax=[]  DOutMin=[]  DOutMax=[]  NOutMin=[]  NOutMax=[]  bOutMin=[]  bOutMax=[]  cOutMin=[]  cOutMax=[]  KbOutMin=[]  KbOutMax=[]  KtOutMin=[]  KtOutMax=[]  IntegratorOutMin=[]  IntegratorOutMax=[]  FilterOutMin=[]  FilterOutMax=[]  SumOutMin=[]  SumOutMax=[]  Sum1OutMin=[]  Sum1OutMax=[]  Sum2OutMin=[]  Sum2OutMax=[]  Sum3OutMin=[]  Sum3OutMax=[]  SumI1OutMin=[]  SumI1OutMax=[]  SumI2OutMin=[]  SumI2OutMax=[]  SumI3OutMin=[]  SumI3OutMax=[]  SumDOutMin=[]  SumDOutMax=[]  SaturationOutMin=[]  SaturationOutMax=[]  IntegratorContinuousStateAttributes=''  IntegratorStateMustResolveToSignalObject=off  IntegratorRTWStateStorageClass=Auto  FilterContinuousStateAttributes=''  FilterStateMustResolveToSignalObject=off  FilterRTWStateStorageClass=Auto  DifferentiatorICPrevScaledInput=0  DifferentiatorOutMin=[]  DifferentiatorOutMax=[]  FilterDiffOutCoefMin=[]  FilterDiffOutCoefMax=[]  SumDenOutMin=[]  SumDenOutMax=[]  SumNumOutMin=[]  SumNumOutMax=[]  ReciprocalOutMin=[]  ReciprocalOutMax=[]  DivideOutMin=[]  DivideOutMax=[]  TunerSelectOption=Transfer Function Based (PID Tuner App)
  emi_1094 : Outport
  wires:
  emi_1092/1 -> cfblk5/1
  emi_1093/1 -> cfblk5/2
  cfblk5/1 -> emi_1094/1

== system sampleModel7293_pp_1_1/cfblk184/cfblk16/cfblk6 ==
  emi_257 : Inport
  Action Port : ActionPort  ActionType=then
  cfblk6 : DiscreteIntegrator  SampleTime=-1  OutDataTypeStr=double  ICPrevOutput=DiscIntNeverNeededParam  ICPrevScaledInput=DiscIntNeverNeededParam
  emi_258 : Outport
  wires:
  emi_257/1 -> cfblk6/1
  cfblk6/1 -> emi_258/1

== system sampleModel7293_pp_1_1/cfblk184/cfblk16/emi_1003 ==
  Action Port : ActionPort  ActionType=else
  emi_1004 : Assertion

== system sampleModel7293_pp_1_1/cfblk184/cfblk16/emi_1066 ==
  Action Port : ActionPort  ActionType=else
  emi_1067 : Assertion

== system sampleModel7293_pp_1_1/cfblk184/cfblk16/emi_1095 ==
  Action Port : ActionPort  ActionType=else
  emi_1096 : Assertion

== system sampleModel7293_pp_1_1/cfblk184/cfblk16/emi_259 ==
  Action Port : ActionPort  ActionType=else
  emi_260 : Assertion

== system sampleModel7293_pp_1_1/cfblk184/cfblk16/emi_410 ==
  Action Port : ActionPort  ActionType=else
  emi_411 : Assertion

== system sampleModel7293_pp_1_1/cfblk184/cfblk17/cfblk14 ==
  emi_1920 : Inport
  Action Port : ActionPort  ActionType=then
  cfblk14 : DiscreteZeroPole  Poles=[0 0.5]  Gain=1  SampleTime=-1
  emi_1921 : Outport
  wires:
  emi_1920/1 -> cfblk14/1
  cfblk14/1 -> emi_1921/1

== system sampleModel7293_pp_1_1/cfblk184/cfblk17/cfblk8 ==
  emi_938 : Inport
  Action Port : ActionPort  ActionType=then
  cfblk8 : DiscreteFilter
  emi_939 : Outport
  wires:
  emi_938/1 -> cfblk8/1
  cfblk8/1 -> emi_939/1

== system sampleModel7293_pp_1_1/cfblk184/cfblk17/cfblk9 ==
  emi_1202 : Inport
  Action Port : ActionPort  ActionType=then
  cfblk9 : Delay
  emi_1203 : Outport
  wires:
  emi_1202/1 -> cfblk9/1
  cfblk9/1 -> emi_1203/1

== system sampleModel7293_pp_1_1/cfblk184/cfblk17/emi_1204 ==
  Action Port : ActionPort  ActionType=else
  emi_1205 : Assertion

== system sampleModel7293_pp_1_1/cfblk184/cfblk17/emi_1922 ==
  Action Port : ActionPort  ActionType=else
  emi_1923 : Assertion

== system sampleModel7293_pp_1_1/cfblk184/cfblk17/emi_940 ==
  Action Port : ActionPort  ActionType=else
  emi_941 : Assertion

== system sampleModel7293_pp_1_1/cfblk185/cfblk18/cfblk4 ==
  emi_1828 : Inport
  emi_1829 : Inport  Port=2
  Action Port : ActionPort  ActionType=then
  cfblk4 : simulink/Continuous/PID Controller (2DOF)  Controller=PID  TimeDomain=Discrete-time  SampleTime=-1  IntegratorMethod=Forward Euler  FilterMethod=Forward Euler  Form=Parallel  UseFilter=on  ControllerParametersSource=internal  P=1  I=1  D=0  N=100  b=1  c=1  InitialConditionSource=internal  InitialConditionForIntegrator=0  InitialConditionForFilter=0  ExternalReset=none  LimitOutput=off  UpperSaturationLimit=inf  LowerSaturationLimit=-inf  LinearizeAsGain=off  AntiWindupMode=none  Kb=1  TrackingMode=off  Kt=1  PParamMin=[]  PParamMax=[]  IParamMin=[]  IParamMax=[]  DParamMin=[]  DParamMax=[]  NParamMin=[]  NParamMax=[]  bParamMin=[]  bParamMax=[]  cParamMin=[]  cParamMax=[]  KbParamMin=[]  KbParamMax=[]  KtParamMin=[]  KtParamMax=[]  POutMin=[]  POutMax=[]  IOutMin=[]  IOutMax=[]  DOutMin=[]  DOutMax=[]  NOutMin=[]  NOutMax=[]  bOutMin=[]  bOutMax=[]  cOutMin=[]  cOutMax=[]  KbOutMin=[]  KbOutMax=[]  KtOutMin=[]  KtOutMax=[]  IntegratorOutMin=[]  IntegratorOutMax=[]  FilterOutMin=[]  FilterOutMax=[]  SumOutMin=[]  SumOutMax=[]  Sum1OutMin=[]  Sum1OutMax=[]  Sum2OutMin=[]  Sum2OutMax=[]  Sum3OutMin=[]  Sum3OutMax=[]  SumI1OutMin=[]  SumI1OutMax=[]  SumI2OutMin=[]  SumI2OutMax=[]  SumI3OutMin=[]  SumI3OutMax=[]  SumDOutMin=[]  SumDOutMax=[]  SaturationOutMin=[]  SaturationOutMax=[]  IntegratorContinuousStateAttributes=''  IntegratorStateMustResolveToSignalObject=off  IntegratorRTWStateStorageClass=Auto  FilterContinuousStateAttributes=''  FilterStateMustResolveToSignalObject=off  FilterRTWStateStorageClass=Auto  DifferentiatorICPrevScaledInput=0  DifferentiatorOutMin=[]  DifferentiatorOutMax=[]  FilterDiffOutCoefMin=[]  FilterDiffOutCoefMax=[]  SumDenOutMin=[]  SumDenOutMax=[]  SumNumOutMin=[]  SumNumOutMax=[]  ReciprocalOutMin=[]  ReciprocalOutMax=[]  DivideOutMin=[]  DivideOutMax=[]  TunerSelectOption=Transfer Function Based (PID Tuner App)
  emi_1830 : Outport
  wires:
  emi_1828/1 -> cfblk4/1
  emi_1829/1 -> cfblk4/2
  cfblk4/1 -> emi_1830/1

== system sampleModel7293_pp_1_1/cfblk185/cfblk18/cfblk5 ==
  emi_653 : Inport
  Action Port : ActionPort  ActionType=then
  cfblk5 : DiscreteFir
  emi_654 : Outport
  wires:
  emi_653/1 -> cfblk5/1
  cfblk5/1 -> emi_654/1

== system sampleModel7293_pp_1_1/cfblk185/cfblk18/emi_1831 ==
  Action Port : ActionPort  ActionType=else
  emi_1832 : Assertion

== system sampleModel7293_pp_1_1/cfblk185/cfblk18/emi_655 ==
  Action Port : ActionPort  ActionType=else
  emi_656 : Assertion

== system sampleModel7293_pp_1_1/cfblk185/cfblk19/cfblk4 ==
  emi_1756 : Inport
  emi_1757 : Inport  Port=2
  Action Port : ActionPort  ActionType=then
  cfblk4 : simulink/Continuous/PID Controller (2DOF)  Controller=PID  TimeDomain=Discrete-time  SampleTime=-1  IntegratorMethod=Forward Euler  FilterMethod=Forward Euler  Form=Parallel  UseFilter=on  ControllerParametersSource=internal  P=1  I=1  D=0  N=100  b=1  c=1  InitialConditionSource=internal  InitialConditionForIntegrator=0  InitialConditionForFilter=0  ExternalReset=none  LimitOutput=off  UpperSaturationLimit=inf  LowerSaturationLimit=-inf  LinearizeAsGain=off  AntiWindupMode=none  Kb=1  TrackingMode=off  Kt=1  PParamMin=[]  PParamMax=[]  IParamMin=[]  IParamMax=[]  DParamMin=[]  DParamMax=[]  NParamMin=[]  NParamMax=[]  bParamMin=[]  bParamMax=[]  cParamMin=[]  cParamMax=[]  KbParamMin=[]  KbParamMax=[]  KtParamMin=[]  KtParamMax=[]  POutMin=[]  POutMax=[]  IOutMin=[]  IOutMax=[]  DOutMin=[]  DOutMax=[]  NOutMin=[]  NOutMax=[]  bOutMin=[]  bOutMax=[]  cOutMin=[]  cOutMax=[]  KbOutMin=[]  KbOutMax=[]  KtOutMin=[]  KtOutMax=[]  IntegratorOutMin=[]  IntegratorOutMax=[]  FilterOutMin=[]  FilterOutMax=[]  SumOutMin=[]  SumOutMax=[]  Sum1OutMin=[]  Sum1OutMax=[]  Sum2OutMin=[]  Sum2OutMax=[]  Sum3OutMin=[]  Sum3OutMax=[]  SumI1OutMin=[]  SumI1OutMax=[]  SumI2OutMin=[]  SumI2OutMax=[]  SumI3OutMin=[]  SumI3OutMax=[]  SumDOutMin=[]  SumDOutMax=[]  SaturationOutMin=[]  SaturationOutMax=[]  IntegratorContinuousStateAttributes=''  IntegratorStateMustResolveToSignalObject=off  IntegratorRTWStateStorageClass=Auto  FilterContinuousStateAttributes=''  FilterStateMustResolveToSignalObject=off  FilterRTWStateStorageClass=Auto  DifferentiatorICPrevScaledInput=0  DifferentiatorOutMin=[]  DifferentiatorOutMax=[]  FilterDiffOutCoefMin=[]  FilterDiffOutCoefMax=[]  SumDenOutMin=[]  SumDenOutMax=[]  SumNumOutMin=[]  SumNumOutMax=[]  ReciprocalOutMin=[]  ReciprocalOutMax=[]  DivideOutMin=[]  DivideOutMax=[]  TunerSelectOption=Transfer Function Based (PID Tuner App)
  emi_1758 : Outport
  wires:
  emi_1756/1 -> cfblk4/1
  emi_1757/1 -> cfblk4/2
  cfblk4/1 -> emi_1758/1

== system sampleModel7293_pp_1_1/cfblk185/cfblk19/cfblk7 ==
  emi_1379 : Inport
  Action Port : ActionPort  ActionType=then
  cfblk7 : Delay
  emi_1380 : Outport
  wires:
  emi_1379/1 -> cfblk7/1
  cfblk7/1 -> emi_1380/1

== system sampleModel7293_pp_1_1/cfblk185/cfblk19/emi_1381 ==
  Action Port : ActionPort  ActionType=else
  emi_1382 : Assertion

== system sampleModel7293_pp_1_1/cfblk185/cfblk19/emi_1759 ==
  Action Port : ActionPort  ActionType=else
  emi_1760 : Assertion

== system sampleModel7293_pp_1_1/cfblk187/cfblk11/cfblk12 ==
  emi_1351 : Inport
  Action Port : ActionPort  ActionType=then
  cfblk12 : simulink/Discrete/Transfer Fcn Real Zero  ZeroZ=0.75  ICPrevInput=0.0  DoSatur=off
      settings: SourceProductName=Simulink  SourceProductBaseCode=SL
  emi_1352 : Outport
  wires:
  emi_1351/1 -> cfblk12/1
  cfblk12/1 -> emi_1352/1

== system sampleModel7293_pp_1_1/cfblk187/cfblk11/cfblk15 ==
  emi_718 : Inport
  Action Port : ActionPort  ActionType=then
  cfblk15 : Delay
  emi_719 : Outport
  wires:
  emi_718/1 -> cfblk15/1
  cfblk15/1 -> emi_719/1

== system sampleModel7293_pp_1_1/cfblk187/cfblk11/cfblk3 ==
  emi_2005 : Inport
  Action Port : ActionPort  ActionType=then
  cfblk3 : DiscreteStateSpace  SampleTime=-1
  emi_2006 : Outport
  wires:
  emi_2005/1 -> cfblk3/1
  cfblk3/1 -> emi_2006/1

== system sampleModel7293_pp_1_1/cfblk187/cfblk11/cfblk9 ==
  emi_1536 : Inport
  Action Port : ActionPort  ActionType=then
  cfblk9 : DiscreteZeroPole  Poles=[0 0.5]  Gain=1  SampleTime=-1
  emi_1537 : Outport
  wires:
  emi_1536/1 -> cfblk9/1
  cfblk9/1 -> emi_1537/1

== system sampleModel7293_pp_1_1/cfblk187/cfblk11/emi_1353 ==
  Action Port : ActionPort  ActionType=else
  emi_1354 : Assertion

== system sampleModel7293_pp_1_1/cfblk187/cfblk11/emi_1538 ==
  Action Port : ActionPort  ActionType=else
  emi_1539 : Assertion

== system sampleModel7293_pp_1_1/cfblk187/cfblk11/emi_2007 ==
  Action Port : ActionPort  ActionType=else
  emi_2008 : Assertion

== system sampleModel7293_pp_1_1/cfblk187/cfblk11/emi_720 ==
  Action Port : ActionPort  ActionType=else
  emi_721 : Assertion
